simulink model "Simscape_Actuated_Robot"  (R2025b)
settings: Solver=odeN  StartTime=0.0  StopTime=20  RelTol=1e-1  AbsTol=1e-3
InitFcn:
  | run("init.m");
values from neighbouring files (symbols this model uses):
  B = [0 1 0; 1 0 0; 0 0 1; 0 0 0]    [init.m]
  q_init = zeros(6,1)    [init.m]
  s = de + c.*e    [wbr_ctrl.m]
  Ts = 1e-4    (= 0.0001)    [init.m]
undefined symbols (not defined in the file or in its folder): K, robot_params, X, Y, Z
libraries: nesl_utility x53, sm_lib x52, simulink x1
(part 1 of 2)
settings Model: Creator=Acer  LastModifiedBy=Acer
settings SolverCC: AutoScaleAbsTol=off  ODENIntegrationMethod=ode8

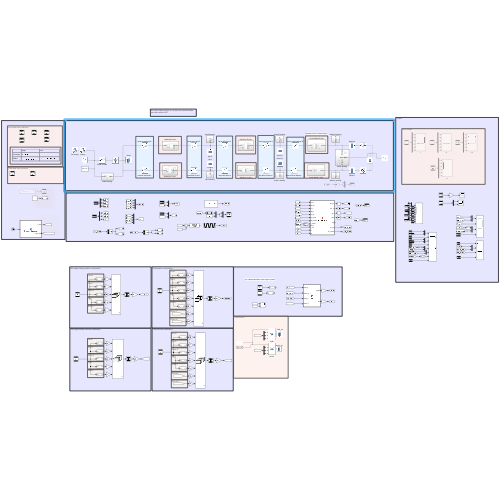
[thumbnail: Simulink's stored preview of the top-level diagram]
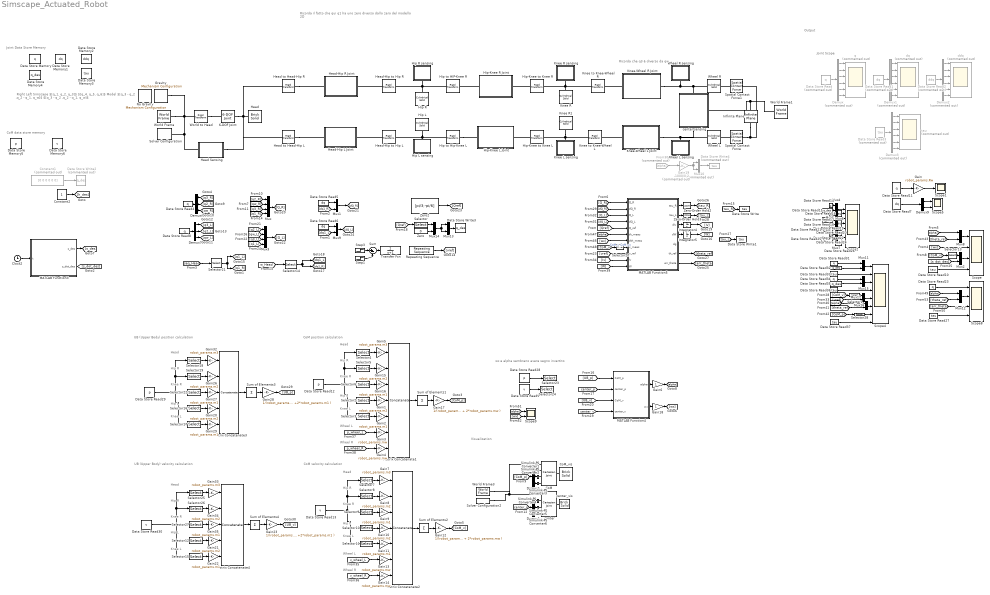
== system Simscape_Actuated_Robot ==
  note: Ricorda che q3 è diverso da qw
  note: wx e alpha sembrano avere segno invertito
  note: Visualization
  note: CoM data store memory
  note: CoM position calculation
  note: ​
      | Right
      | Left
      |
      | Simscape
      | $[q_1, q_2, q_3]$
      | $[q_4, q_5, q_6]$
      |
      | Model
      | $[q_3 - q_2 ,q_2 - q_1, q_w]$
      | $[q_3 - q_2 ,q_2 - q_1, q_w]$
  note: Joint Data Store Memory
  note: Joint Scope
  note: Output
  note: Ricorda il fatto che qui q1 ha uno zero diverso dallo
      | zero del modello 2D
  note: Head
  note: CoM velocity calculation
  note: Hip R
  note: Knee R
  note: Hip L
  note: Knee L
  note: Wheel L
  note: Wheel R
  note: Wheel L
  note: Wheel R
  note: Head
  note: Knee L
  note: Hip R
  note: Knee R
  note: Hip L
  note: UB (Upper Body) position calculation
  note: Head
  note: UB (Upper Body) velocity calculation
  note: Hip R
  note: Knee R
  note: Hip L
  note: Knee L
  note: Head
  note: Knee L
  note: Hip R
  note: Knee R
  note: Hip L
  6-DOF Joint : sm_lib/Joints/6-DOF Joint  JointMode=Normal  CompositeWrenchDir=FollowerOnBase  CompositeWrenchFrame=BaseFrame  SenseConstraintForce=off  SenseConstraintTorque=off  SenseTotalForce=off  SenseTotalTorque=off  PxPositionTargetSpecify=off  PxPositionTargetPriority=High  PxPositionTargetValue=0  PxPositionTargetValueUnits=m  PxVelocityTargetSpecify=off  PxVelocityTargetPriority=High  PxVelocityTargetValue=0  PxVelocityTargetValueUnits=m/s  PxEquilibriumPosition=0  PxEquilibriumPositionUnits=m  PxSpringStiffness=0  PxSpringStiffnessUnits=N/m  PxDampingCoefficient=0  PxDampingCoefficientUnits=N/(m/s)  PxLowerLimitSpecify=off  PxLowerLimitBound=-1  PxLowerLimitBoundUnits=m  PxLowerLimitStiffness=1e6  PxLowerLimitStiffnessUnits=N/m  PxLowerLimitDamping=1e3  PxLowerLimitDampingUnits=N/(m/s)  PxLowerLimitTransitionRegionWidth=1e-4  PxLowerLimitTransitionRegionWidthUnits=m  PxUpperLimitSpecify=off  PxUpperLimitBound=1  PxUpperLimitBoundUnits=m  PxUpperLimitStiffness=1e6  PxUpperLimitStiffnessUnits=N/m  PxUpperLimitDamping=1e3  PxUpperLimitDampingUnits=N/(m/s)  PxUpperLimitTransitionRegionWidth=1e-4  PxUpperLimitTransitionRegionWidthUnits=m  PxTorqueActuationMode=NoTorque  PxMotionActuationMode=ComputedMotion  PxSensePosition=off  PxSenseVelocity=off  PxSenseAcceleration=off  PxSenseTorqueForce=off  PxSenseLowerLimitTorqueForce=off  PxSenseUpperLimitTorqueForce=off  PyPositionTargetSpecify=off  PyPositionTargetPriority=High  PyPositionTargetValue=0  PyPositionTargetValueUnits=m  PyVelocityTargetSpecify=off  PyVelocityTargetPriority=High  PyVelocityTargetValue=0  PyVelocityTargetValueUnits=m/s  PyEquilibriumPosition=0  PyEquilibriumPositionUnits=m  PySpringStiffness=0  PySpringStiffnessUnits=N/m  PyDampingCoefficient=0  PyDampingCoefficientUnits=N/(m/s)  PyLowerLimitSpecify=off  PyLowerLimitBound=-1  PyLowerLimitBoundUnits=m  PyLowerLimitStiffness=1e6  PyLowerLimitStiffnessUnits=N/m  PyLowerLimitDamping=1e3  PyLowerLimitDampingUnits=N/(m/s)  PyLowerLimitTransitionRegionWidth=1e-4  PyLowerLimitTransitionRegionWidthUnits=m  PyUpperLimitSpecify=off  PyUpperLimitBound=1  PyUpperLimitBoundUnits=m  PyUpperLimitStiffness=1e6  PyUpperLimitStiffnessUnits=N/m  PyUpperLimitDamping=1e3  PyUpperLimitDampingUnits=N/(m/s)  PyUpperLimitTransitionRegionWidth=1e-4  PyUpperLimitTransitionRegionWidthUnits=m  PyTorqueActuationMode=NoTorque  PyMotionActuationMode=ComputedMotion  PySensePosition=off  PySenseVelocity=off  PySenseAcceleration=off  PySenseTorqueForce=off  PySenseLowerLimitTorqueForce=off  PySenseUpperLimitTorqueForce=off  PzPositionTargetSpecify=off  PzPositionTargetPriority=High  PzPositionTargetValue=0  PzPositionTargetValueUnits=m  PzVelocityTargetSpecify=off  PzVelocityTargetPriority=High  PzVelocityTargetValue=0  PzVelocityTargetValueUnits=m/s  PzEquilibriumPosition=0  PzEquilibriumPositionUnits=m  PzSpringStiffness=0  PzSpringStiffnessUnits=N/m  PzDampingCoefficient=0  PzDampingCoefficientUnits=N/(m/s)  PzLowerLimitSpecify=off  PzLowerLimitBound=-1  PzLowerLimitBoundUnits=m  PzLowerLimitStiffness=1e6  PzLowerLimitStiffnessUnits=N/m  PzLowerLimitDamping=1e3  PzLowerLimitDampingUnits=N/(m/s)  PzLowerLimitTransitionRegionWidth=1e-4  PzLowerLimitTransitionRegionWidthUnits=m  PzUpperLimitSpecify=off  PzUpperLimitBound=1  PzUpperLimitBoundUnits=m  PzUpperLimitStiffness=1e6  PzUpperLimitStiffnessUnits=N/m  PzUpperLimitDamping=1e3  PzUpperLimitDampingUnits=N/(m/s)  PzUpperLimitTransitionRegionWidth=1e-4  PzUpperLimitTransitionRegionWidthUnits=m  PzTorqueActuationMode=NoTorque  PzMotionActuationMode=ComputedMotion  PzSensePosition=off  PzSenseVelocity=off  PzSenseAcceleration=off  PzSenseTorqueForce=off  PzSenseLowerLimitTorqueForce=off  PzSenseUpperLimitTorqueForce=off  SphPositionTargetSpecify=off  SphPositionTargetPriority=High  SphPositionTargetRotationMethod=None  SphPositionTargetFollAlignAxisA=+X  SphPositionTargetBaseAlignAxisA=+Y  SphPositionTargetFollAlignAxisB=+Y  SphPositionTargetBaseAlignAxisB=+Z  SphPositionTargetRotationStandardAxis=+Z  SphPositionTargetRotationAngle=0  SphPositionTargetRotationAngleUnits=deg  SphPositionTargetRotationArbitraryAxis=[0 0 1]  SphPositionTargetRotationSequenceAxes=FollowerAxes  SphPositionTargetRotationSequence=XYX  SphPositionTargetRotationSequenceAngles=[0 0 0]  SphPositionTargetRotationSequenceAnglesUnits=deg  SphPositionTargetRotationMatrix=[1 0 0;0 1 0;0 0 1]  SphPositionTargetQuaternion=[1 0 0 0]  SphVelocityTargetSpecify=off  SphVelocityTargetPriority=High  SphVelocityTargetValue=[0 0 0]  SphVelocityTargetValueUnits=deg/s  SphVelocityTargetInFollowerFrame=on  SphEqPosRotationMethod=None  SphEqPosFollAlignAxisA=+X  SphEqPosBaseAlignAxisA=+Y  SphEqPosFollAlignAxisB=+Y  SphEqPosBaseAlignAxisB=+Z  SphEqPosRotationStandardAxis=+Z  SphEqPosRotationAngle=0  SphEqPosRotationAngleUnits=deg  SphEqPosRotationArbitraryAxis=[0 0 1]  SphEqPosRotationSequenceAxes=FollowerAxes  SphEqPosRotationSequence=XYX  SphEqPosRotationSequenceAngles=[0 0 0]  SphEqPosRotationSequenceAnglesUnits=deg  SphEqPosRotationMatrix=[1 0 0;0 1 0;0 0 1]  SphEqPosQuaternion=[1 0 0 0]  SphSpringStiffness=0  SphSpringStiffnessUnits=N*m/deg  SphDampingCoefficient=0  SphDampingCoefficientUnits=N*m/(deg/s)  SphLowerLimitSpecify=off  SphLowerLimitBound=15  SphLowerLimitBoundUnits=deg  SphLowerLimitStiffness=1e4  SphLowerLimitStiffnessUnits=N*m/deg  SphLowerLimitDamping=10  SphLowerLimitDampingUnits=N*m/(deg/s)  SphLowerLimitTransitionRegionWidth=0.1  SphLowerLimitTransitionRegionWidthUnits=deg  SphUpperLimitSpecify=off  SphUpperLimitBound=45  SphUpperLimitBoundUnits=deg  SphUpperLimitStiffness=1e4  SphUpperLimitStiffnessUnits=N*m/deg  SphUpperLimitDamping=10  SphUpperLimitDampingUnits=N*m/(deg/s)  SphUpperLimitTransitionRegionWidth=0.1  SphUpperLimitTransitionRegionWidthUnits=deg  SphTorqueActuationMode=NoTorque  SphActuateTorqueX=off  SphActuateTorqueY=off  SphActuateTorqueZ=off  SphActuateTorque=off  SphActuationFrame=BaseFrame  SphSensePosition=off  SphSenseVelocityX=off  SphSenseVelocityY=off  SphSenseVelocityZ=off  SphSenseVelocity=off  SphSenseAccelerationX=off  SphSenseAccelerationY=off  SphSenseAccelerationZ=off  SphSenseAcceleration=off  SphSenseLowerLimitTorqueMag=off  SphSenseUpperLimitTorqueMag=off  SphSensingFrame=BaseFrame
  Clock2 : Clock
  CoM : sm_lib/Joints/Cartesian Joint  JointMode=Normal  CompositeWrenchDir=FollowerOnBase  CompositeWrenchFrame=BaseFrame  SenseConstraintForce=off  SenseConstraintTorque=off  SenseTotalForce=off  SenseTotalTorque=off  PxPositionTargetSpecify=off  PxPositionTargetPriority=High  PxPositionTargetValue=0  PxPositionTargetValueUnits=m  PxVelocityTargetSpecify=off  PxVelocityTargetPriority=High  PxVelocityTargetValue=0  PxVelocityTargetValueUnits=m/s  PxEquilibriumPosition=0  PxEquilibriumPositionUnits=m  PxSpringStiffness=0  PxSpringStiffnessUnits=N/m  PxDampingCoefficient=0  PxDampingCoefficientUnits=N/(m/s)  PxLowerLimitSpecify=off  PxLowerLimitBound=-1  PxLowerLimitBoundUnits=m  PxLowerLimitStiffness=1e6  PxLowerLimitStiffnessUnits=N/m  PxLowerLimitDamping=1e3  PxLowerLimitDampingUnits=N/(m/s)  PxLowerLimitTransitionRegionWidth=1e-4  PxLowerLimitTransitionRegionWidthUnits=m  PxUpperLimitSpecify=off  PxUpperLimitBound=1  PxUpperLimitBoundUnits=m  PxUpperLimitStiffness=1e6  PxUpperLimitStiffnessUnits=N/m  PxUpperLimitDamping=1e3  PxUpperLimitDampingUnits=N/(m/s)  PxUpperLimitTransitionRegionWidth=1e-4  PxUpperLimitTransitionRegionWidthUnits=m  PxTorqueActuationMode=ComputedTorque  PxMotionActuationMode=InputMotion  PxSensePosition=off  PxSenseVelocity=off  PxSenseAcceleration=off  PxSenseTorqueForce=off  PxSenseLowerLimitTorqueForce=off  PxSenseUpperLimitTorqueForce=off  PyPositionTargetSpecify=off  PyPositionTargetPriority=High  PyPositionTargetValue=0  PyPositionTargetValueUnits=m  PyVelocityTargetSpecify=off  PyVelocityTargetPriority=High  PyVelocityTargetValue=0  PyVelocityTargetValueUnits=m/s  PyEquilibriumPosition=0  PyEquilibriumPositionUnits=m  PySpringStiffness=0  PySpringStiffnessUnits=N/m  PyDampingCoefficient=0  PyDampingCoefficientUnits=N/(m/s)  PyLowerLimitSpecify=off  PyLowerLimitBound=-1  PyLowerLimitBoundUnits=m  PyLowerLimitStiffness=1e6  PyLowerLimitStiffnessUnits=N/m  PyLowerLimitDamping=1e3  PyLowerLimitDampingUnits=N/(m/s)  PyLowerLimitTransitionRegionWidth=1e-4  PyLowerLimitTransitionRegionWidthUnits=m  PyUpperLimitSpecify=off  PyUpperLimitBound=1  PyUpperLimitBoundUnits=m  PyUpperLimitStiffness=1e6  PyUpperLimitStiffnessUnits=N/m  PyUpperLimitDamping=1e3  PyUpperLimitDampingUnits=N/(m/s)  PyUpperLimitTransitionRegionWidth=1e-4  PyUpperLimitTransitionRegionWidthUnits=m  PyTorqueActuationMode=ComputedTorque  PyMotionActuationMode=InputMotion  PySensePosition=off  PySenseVelocity=off  PySenseAcceleration=off  PySenseTorqueForce=off  PySenseLowerLimitTorqueForce=off  PySenseUpperLimitTorqueForce=off  PzPositionTargetSpecify=off  PzPositionTargetPriority=High  PzPositionTargetValue=0  PzPositionTargetValueUnits=m  PzVelocityTargetSpecify=off  PzVelocityTargetPriority=High  PzVelocityTargetValue=0  PzVelocityTargetValueUnits=m/s  PzEquilibriumPosition=0  PzEquilibriumPositionUnits=m  PzSpringStiffness=0  PzSpringStiffnessUnits=N/m  PzDampingCoefficient=0  PzDampingCoefficientUnits=N/(m/s)  PzLowerLimitSpecify=off  PzLowerLimitBound=-1  PzLowerLimitBoundUnits=m  PzLowerLimitStiffness=1e6  PzLowerLimitStiffnessUnits=N/m  PzLowerLimitDamping=1e3  PzLowerLimitDampingUnits=N/(m/s)  PzLowerLimitTransitionRegionWidth=1e-4  PzLowerLimitTransitionRegionWidthUnits=m  PzUpperLimitSpecify=off  PzUpperLimitBound=1  PzUpperLimitBoundUnits=m  PzUpperLimitStiffness=1e6  PzUpperLimitStiffnessUnits=N/m  PzUpperLimitDamping=1e3  PzUpperLimitDampingUnits=N/(m/s)  PzUpperLimitTransitionRegionWidth=1e-4  PzUpperLimitTransitionRegionWidthUnits=m  PzTorqueActuationMode=ComputedTorque  PzMotionActuationMode=InputMotion  PzSensePosition=off  PzSenseVelocity=off  PzSenseAcceleration=off  PzSenseTorqueForce=off  PzSenseLowerLimitTorqueForce=off  PzSenseUpperLimitTorqueForce=off
  CoM_vis : sm_lib/Body Elements/Brick Solid  BrickDimensions=[.05 .05 .05]  BrickDimensionsUnits=m  ExportEntireGeometry=off  InertiaType=PointMass  BasedOnType=Density  Density=1000  DensityUnits=kg/m^3  Mass=0.001  MassUnits=kg  CenterOfMass=[0 0 0]  CenterOfMassUnits=m  MomentsOfInertia=[1 1 1]  MomentsOfInertiaUnits=kg*m^2  ProductsOfInertia=[0 0 0]  ProductsOfInertiaUnits=kg*m^2  GraphicType=FromGeometry  MarkerShape=Sphere  MarkerSize=10  GraphicVisPropType=SimpleVisualProperties  GraphicDiffuseColor=[0 0 0]  GraphicOpacity=1  GraphicSpecularColor=[0.5 0.5 0.5 1.0]  GraphicAmbientColor=[0.15 0.15 0.15 1.0]  GraphicEmissiveColor=[0.0 0.0 0.0 1.0]  GraphicShininess=75  DoExposeReferenceFrame=on  SerializedFrames=<Frames/>
  Constant1 : Constant  Commented=on  Value=[0 0 0 0 0 0]
  Constant2 : Constant
  Data Store Memory : DataStoreMemory  Priority=1  DataStoreName=q  WriteAfterWriteMsg=warning  InitialValue=q_init  ShareAcrossModelInstances=on  ShowAdditionalParam=off  OutDataTypeStr=double
  Data Store Memory1 : DataStoreMemory  Priority=2  DataStoreName=dq  WriteAfterWriteMsg=warning  InitialValue=zeros(6,1)  ShareAcrossModelInstances=on  ShowAdditionalParam=off  OutDataTypeStr=double
  Data Store Memory2 : DataStoreMemory  Priority=2  DataStoreName=ddq  WriteAfterWriteMsg=warning  InitialValue=zeros(6,1)  ShareAcrossModelInstances=on  ShowAdditionalParam=off  OutDataTypeStr=double
  Data Store Memory3 : DataStoreMemory  Priority=2  DataStoreName=tau  WriteAfterWriteMsg=warning  InitialValue=zeros(6,1)  ShareAcrossModelInstances=on  ShowAdditionalParam=off  OutDataTypeStr=double
  Data Store Memory4 : DataStoreMemory  DataStoreName=q_des  WriteAfterWriteMsg=warning  InitialValue=zeros(6,1)  ShareAcrossModelInstances=on  ShowAdditionalParam=off  OutDataTypeStr=double
  Data Store Memory5 : DataStoreMemory  Priority=2  DataStoreName=p  WriteAfterWriteMsg=warning  InitialValue=zeros(3,5)  ShareAcrossModelInstances=on  ShowAdditionalParam=off  OutDataTypeStr=double
  Data Store Memory6 : DataStoreMemory  Priority=2  DataStoreName=v  WriteAfterWriteMsg=warning  InitialValue=zeros(3,5)  ShareAcrossModelInstances=on  ShowAdditionalParam=off  OutDataTypeStr=double
  Data Store Read : DataStoreRead  Commented=on  DataStoreName=q  IndexOptions=Index vector (dialog)  Indices=1  OutputSizes=1
  Data Store Read1 : DataStoreRead  Commented=on  DataStoreName=dq  IndexOptions=Index vector (dialog)  Indices=1  OutputSizes=1
  Data Store Read10 : DataStoreRead  DataStoreName=tau  DataStoreElements=tau  EnableIndexing=on  IndexOptions=Index vector (dialog)  Indices=[3 6]  OutputSizes=1
  Data Store Read11 : DataStoreRead  DataStoreName=q  DataStoreElements=q  EnableIndexing=on  IndexOptions=Index vector (dialog)  Indices=[3]  OutputSizes=1
  Data Store Read12 : DataStoreRead  DataStoreName=p  IndexOptions=Index vector (dialog)  Indices=1  OutputSizes=1
  Data Store Read13 : DataStoreRead  DataStoreName=v  IndexOptions=Index vector (dialog)  Indices=1  OutputSizes=1
  Data Store Read14 : DataStoreRead  DataStoreName=q  DataStoreElements=q  EnableIndexing=on  IndexOptions=Index vector (dialog)  Indices=1  OutputSizes=1
  Data Store Read15 : DataStoreRead  DataStoreName=q_des  DataStoreElements=q_des  EnableIndexing=on  IndexOptions=Index vector (dialog)  Indices=[1]  OutputSizes=1
  Data Store Read16 : DataStoreRead  DataStoreName=tau  DataStoreElements=tau  EnableIndexing=on  IndexOptions=Index vector (dialog)  Indices=1  OutputSizes=1
  Data Store Read17 : DataStoreRead  DataStoreName=q  DataStoreElements=q  EnableIndexing=on  IndexOptions=Index vector (dialog)  Indices=2  OutputSizes=1
  Data Store Read18 : DataStoreRead  DataStoreName=q_des  DataStoreElements=q_des  EnableIndexing=on  IndexOptions=Index vector (dialog)  Indices=[2]  OutputSizes=1
  Data Store Read19 : DataStoreRead  DataStoreName=tau  DataStoreElements=tau  EnableIndexing=on  IndexOptions=Index vector (dialog)  Indices=2  OutputSizes=1
  Data Store Read2 : DataStoreRead  Commented=on  DataStoreName=ddq  IndexOptions=Index vector (dialog)  Indices=1  OutputSizes=1
  Data Store Read20 : DataStoreRead  DataStoreName=q  DataStoreElements=q  EnableIndexing=on  IndexOptions=Index vector (dialog)  Indices=4  OutputSizes=1
  Data Store Read21 : DataStoreRead  DataStoreName=q_des  DataStoreElements=q_des  EnableIndexing=on  IndexOptions=Index vector (dialog)  Indices=4  OutputSizes=1
  Data Store Read22 : DataStoreRead  DataStoreName=tau  DataStoreElements=tau  EnableIndexing=on  IndexOptions=Index vector (dialog)  Indices=4  OutputSizes=1
  Data Store Read23 : DataStoreRead  DataStoreName=q  EnableIndexing=on  IndexOptions=Index vector (dialog)  Indices=[3 6]  OutputSizes=1
  Data Store Read24 : DataStoreRead  DataStoreName=q  DataStoreElements=q  EnableIndexing=on  IndexOptions=Index vector (dialog)  Indices=5  OutputSizes=1
  Data Store Read25 : DataStoreRead  DataStoreName=q_des  DataStoreElements=q_des  EnableIndexing=on  IndexOptions=Index vector (dialog)  Indices=5  OutputSizes=1
  Data Store Read26 : DataStoreRead  DataStoreName=tau  DataStoreElements=tau  EnableIndexing=on  IndexOptions=Index vector (dialog)  Indices=5  OutputSizes=1
  Data Store Read27 : DataStoreRead  DataStoreName=tau  DataStoreElements=tau  EnableIndexing=on  IndexOptions=Index vector (dialog)  Indices=[3 6]  OutputSizes=1
  Data Store Read28 : DataStoreRead  DataStoreName=p  IndexOptions=Index vector (dialog)  Indices=1  OutputSizes=1
  Data Store Read29 : DataStoreRead  DataStoreName=p  IndexOptions=Index vector (dialog)  Indices=1  OutputSizes=1
  Data Store Read3 : DataStoreRead  Commented=on  DataStoreName=tau  IndexOptions=Index vector (dialog)  Indices=1  OutputSizes=1
  Data Store Read30 : DataStoreRead  DataStoreName=v  IndexOptions=Index vector (dialog)  Indices=1  OutputSizes=1
  Data Store Read31 : DataStoreRead  DataStoreName=q  DataStoreElements=q  EnableIndexing=on  IndexOptions=Index vector (dialog)  Indices=1  OutputSizes=1
  Data Store Read32 : DataStoreRead  DataStoreName=q_des  DataStoreElements=q_des  EnableIndexing=on  IndexOptions=Index vector (dialog)  Indices=[1]  OutputSizes=1
  Data Store Read33 : DataStoreRead  DataStoreName=tau  DataStoreElements=tau  EnableIndexing=on  IndexOptions=Index vector (dialog)  Indices=1  OutputSizes=1
  Data Store Read34 : DataStoreRead  DataStoreName=q  DataStoreElements=q  EnableIndexing=on  IndexOptions=Index vector (dialog)  Indices=2  OutputSizes=1
  Data Store Read35 : DataStoreRead  DataStoreName=q_des  DataStoreElements=q_des  EnableIndexing=on  IndexOptions=Index vector (dialog)  Indices=[2]  OutputSizes=1
  Data Store Read36 : DataStoreRead  DataStoreName=tau  DataStoreElements=tau  EnableIndexing=on  IndexOptions=Index vector (dialog)  Indices=2  OutputSizes=1
  Data Store Read37 : DataStoreRead  DataStoreName=tau  DataStoreElements=tau  EnableIndexing=on  IndexOptions=Index vector (dialog)  Indices=[3 6]  OutputSizes=1
  Data Store Read4 : DataStoreRead  DataStoreName=q  DataStoreElements=q  EnableIndexing=on  IndexOptions=Index vector (dialog)  Indices=[1 2 3]  OutputSizes=1
  Data Store Read5 : DataStoreRead  DataStoreName=dq  DataStoreElements=dq  EnableIndexing=on  IndexOptions=Index vector (dialog)  Indices=[2 3 1]  OutputSizes=1
  Data Store Read6 : DataStoreRead  DataStoreName=dq  DataStoreElements=dq  EnableIndexing=on  IndexOptions=Index vector (dialog)  Indices=[5 6 4]  OutputSizes=1
  Data Store Read7 : DataStoreRead  DataStoreName=dq  DataStoreElements=dq  EnableIndexing=on  IndexOptions=Index vector (dialog)  Indices=[3, 6]  OutputSizes=1
  Data Store Read8 : DataStoreRead  DataStoreName=q  DataStoreElements=q  EnableIndexing=on  IndexOptions=Index vector (dialog)  Indices=[4 5 6]  OutputSizes=1
  Data Store Read9 : DataStoreRead  DataStoreName=v  IndexOptions=Index vector (dialog)  Indices=1  OutputSizes=1
  Data Store Write : DataStoreWrite  DataStoreName=tau  DataStoreElements=tau  EnableIndexing=on  IndexOptions=Index vector (dialog)  Indices=[3 2 1]  OutputSizes=1
  Data Store Write1 : DataStoreWrite  DataStoreName=tau  DataStoreElements=tau  EnableIndexing=on  IndexOptions=Index vector (dialog)  Indices=[6 5 4]  OutputSizes=1
  Data Store Write2 : DataStoreWrite  Commented=on  DataStoreName=q_des  IndexOptions=Index vector (dialog)  Indices=1  OutputSizes=1
  Data Store Write3 : DataStoreWrite  DataStoreName=q_des  IndexOptions=Index vector (dialog)  Indices=1  OutputSizes=1
  Data Store Write4 : DataStoreWrite  Commented=on  DataStoreName=tau  DataStoreElements=tau  EnableIndexing=on  IndexOptions=Index vector (dialog)  Indices=[3 6]  OutputSizes=1
  Demux{,1..3} (4 alike) : Demux  Commented=on  Outputs=6
  Demux{4..7} (4 alike) : Demux  Outputs=3
  Demux9 : Demux  Outputs=2
  From30 : From  Commented=on  GotoTag=alpha
  Gain : Gain  Gain=robot_params.Rw
  Gain{1,8,10,15,20..21,26,34} (8 alike) : Gain  Gain=robot_params.m2
  Gain{2,9,11,16,22,27,29,35} (8 alike) : Gain  Gain=robot_params.m1
  Gain12 : Gain  Gain=1/(robot_params.m3 + 2*robot_params.m2 +2*robot_params.m1 + 2*robot_params.mw )
  Gain{3..4,13..14} (4 alike) : Gain  Gain=robot_params.mw
  Gain17 : Gain  Gain=1/(robot_params.m3 + 2*robot_params.m2 +2*robot_params.m1 + 2*robot_params.mw )
  Gain18 : Gain
  Gain19 : Gain  Commented=on  Gain=-1000/0.2
  Gain23 : Gain  Gain=1/(robot_params.m3 + 2*robot_params.m2 +2*robot_params.m1 )
  Gain28 : Gain  Gain=1/(robot_params.m3 + 2*robot_params.m2 +2*robot_params.m1 )
  Gain{5,7,32..33} (4 alike) : Gain  Gain=robot_params.m3
  Gain6 : Gain
  Gravity : sm_lib/Utilities/Mechanism Configuration  UniformGravity=Constant  GravityVector=[0 0 -9.80665]  GravityVectorUnits=m/s^2  LinearizationDelta=0.001  JointModeTransitionNonlinearIterations=2
  Head : sm_lib/Body Elements/Brick Solid  BrickDimensions=robot_params.length_torso  BrickDimensionsUnits=m  ExportEntireGeometry=off  InertiaType=Custom  BasedOnType=Density  Density=1000  DensityUnits=kg/m^3  Mass=robot_params.m3  MassUnits=kg  CenterOfMass=[0 0 0]  CenterOfMassUnits=m  MomentsOfInertia=robot_params.inertia_torso  MomentsOfInertiaUnits=kg*m^2  ProductsOfInertia=[0 0 0]  ProductsOfInertiaUnits=kg*m^2  GraphicType=FromGeometry  MarkerShape=Sphere  MarkerSize=10  GraphicVisPropType=SimpleVisualProperties  GraphicDiffuseColor=[0.5 0.5 0.5]  GraphicOpacity=1  GraphicSpecularColor=[0.5 0.5 0.5 1.0]  GraphicAmbientColor=[0.15 0.15 0.15 1.0]  GraphicEmissiveColor=[0.0 0.0 0.0 1.0]  GraphicShininess=75  DoExposeReferenceFrame=on  SerializedFrames=<Frames/>
  Head Sensing : Subsystem
  "Head to Head-Hip L " : sm_lib/Frames and Transforms/Rigid Transform  RotationMethod=RotationSequence  FollAlignAxisA=+X  BaseAlignAxisA=+Y  FollAlignAxisB=+Y  BaseAlignAxisB=+Z  RotationStandardAxis=+Z  RotationAngle=0  RotationAngleUnits=deg  RotationArbitraryAxis=[0 0 1]  RotationSequenceAxes=FollowerAxes  RotationSequence=XYZ  RotationSequenceAngles=[pi/2 0 0]  RotationSequenceAnglesUnits=rad  RotationMatrix=[1 0 0;0 1 0;0 0 1]  Quaternion=[1 0 0 0]  TranslationMethod=Cartesian  TranslationCartesianOffset=[0 -63/2 -35/2]  TranslationCartesianOffsetUnits=cm  TranslationStandardAxis=+Z  TranslationStandardOffset=0  TranslationStandardOffsetUnits=m  TranslationROffset=0  TranslationROffsetUnits=m  TranslationThetaOffset=0  TranslationThetaOffsetUnits=deg  TranslationZOffset=0  TranslationZOffsetUnits=m
  "Head to Head-Hip R  " : sm_lib/Frames and Transforms/Rigid Transform  RotationMethod=RotationSequence  FollAlignAxisA=+X  BaseAlignAxisA=+Y  FollAlignAxisB=+Y  BaseAlignAxisB=+Z  RotationStandardAxis=+Z  RotationAngle=0  RotationAngleUnits=deg  RotationArbitraryAxis=[0 0 1]  RotationSequenceAxes=FollowerAxes  RotationSequence=XYZ  RotationSequenceAngles=[pi/2 0 0]  RotationSequenceAnglesUnits=rad  RotationMatrix=[1 0 0;0 1 0;0 0 1]  Quaternion=[1 0 0 0]  TranslationMethod=Cartesian  TranslationCartesianOffset=[0 63/2 -35/2]  TranslationCartesianOffsetUnits=cm  TranslationStandardAxis=+Z  TranslationStandardOffset=0  TranslationStandardOffsetUnits=m  TranslationROffset=0  TranslationROffsetUnits=m  TranslationThetaOffset=0  TranslationThetaOffsetUnits=deg  TranslationZOffset=0  TranslationZOffsetUnits=m
  "Head-Hip L Joint " : Subsystem
  "Head-Hip R Joint " : Subsystem
  Head-Hip to Hip L : sm_lib/Frames and Transforms/Rigid Transform  RotationMethod=RotationSequence  FollAlignAxisA=+X  BaseAlignAxisA=+Y  FollAlignAxisB=+Y  BaseAlignAxisB=+Z  RotationStandardAxis=+Z  RotationAngle=0  RotationAngleUnits=deg  RotationArbitraryAxis=[0 0 1]  RotationSequenceAxes=FollowerAxes  RotationSequence=XYZ  RotationSequenceAngles=[pi/2 0 0]  RotationSequenceAnglesUnits=rad  RotationMatrix=[1 0 0;0 1 0;0 0 1]  Quaternion=[1 0 0 0]  TranslationMethod=Cartesian  TranslationCartesianOffset=[0 -45/2 0]  TranslationCartesianOffsetUnits=cm  TranslationStandardAxis=+Z  TranslationStandardOffset=0  TranslationStandardOffsetUnits=m  TranslationROffset=0  TranslationROffsetUnits=m  TranslationThetaOffset=0  TranslationThetaOffsetUnits=deg  TranslationZOffset=0  TranslationZOffsetUnits=m
  Head-Hip to Hip R : sm_lib/Frames and Transforms/Rigid Transform  RotationMethod=RotationSequence  FollAlignAxisA=+X  BaseAlignAxisA=+Y  FollAlignAxisB=+Y  BaseAlignAxisB=+Z  RotationStandardAxis=+Z  RotationAngle=0  RotationAngleUnits=deg  RotationArbitraryAxis=[0 0 1]  RotationSequenceAxes=FollowerAxes  RotationSequence=XYZ  RotationSequenceAngles=[pi/2 0 0]  RotationSequenceAnglesUnits=rad  RotationMatrix=[1 0 0;0 1 0;0 0 1]  Quaternion=[1 0 0 0]  TranslationMethod=Cartesian  TranslationCartesianOffset=[0 -45/2 0]  TranslationCartesianOffsetUnits=cm  TranslationStandardAxis=+Z  TranslationStandardOffset=0  TranslationStandardOffsetUnits=m  TranslationROffset=0  TranslationROffsetUnits=m  TranslationThetaOffset=0  TranslationThetaOffsetUnits=deg  TranslationZOffset=0  TranslationZOffsetUnits=m
  Hip L : sm_lib/Body Elements/Cylindrical Solid  CylinderRadius=robot_params.radius_coscia  CylinderRadiusUnits=m  CylinderLength=robot_params.l2  CylinderLengthUnits=m  ExportEntireGeometry=off  InertiaType=Custom  BasedOnType=Density  Density=1000  DensityUnits=kg/m^3  Mass=robot_params.m2  MassUnits=kg  CenterOfMass=[0 0 0]  CenterOfMassUnits=m  MomentsOfInertia=robot_params.inertia_coscia  MomentsOfInertiaUnits=kg*m^2  ProductsOfInertia=[0 0 0]  ProductsOfInertiaUnits=kg*m^2  GraphicType=FromGeometry  MarkerShape=Sphere  MarkerSize=10  GraphicVisPropType=SimpleVisualProperties  GraphicDiffuseColor=[0.102 0 0.502]  GraphicOpacity=1  GraphicSpecularColor=[0.5 0.5 0.5 1.0]  GraphicAmbientColor=[0.15 0.15 0.15 1.0]  GraphicEmissiveColor=[0.0 0.0 0.0 1.0]  GraphicShininess=75  DoExposeReferenceFrame=on  SerializedFrames=<Frames/>
  Hip L sensing : Subsystem
      settings: PortSchema="{\"entries\":[{\"content\":{\"sides\":[{\"content\":{},\"type\":\"ConnectorPlacement.EquallySpacedRectSide\",\"uuid\":\"ea9d79d0-a490-4652-82e6-557e12b0aba5\"},{\"content\":{\"side\":\"RIGHT\"},\"type\":\"ConnectorPlacement.EquallySpacedRectSide\",\"uuid\":\"f32903a1-4d8b-4407-8bbb-547edd3cb5f6\"},{\"content\":{\"side\":\"TOP\"},\"type\":\"ConnectorPlacement.EquallySpacedRectSide\",\"uuid\":\"fbee0b4d-6271-40ea-8dd1-d28f8c19f4ef\"},{\"content\":{\"connectorIds\":[\"RConn1\"],\"side\":\"BOTTOM\"},\"type\":\"ConnectorPlacement.EquallySpacedRectSide\",\"uuid\":\"cbab87b1-08d9-47a6-9493-a07b4ae6b609\"}]},\"type\":\"ConnectorPlacement.EquallySpacedConnector\",\"uuid\":\"a82548d1-a5fc-4c9c-b8a0-1d70df1cc0c8\"}],\"packageUris\":[\"http://schema.mathworks.com/mf0/Connector/R2020b\"],\"version\":\"1.0\"}"
  Hip R : sm_lib/Body Elements/Cylindrical Solid  CylinderRadius=robot_params.radius_coscia  CylinderRadiusUnits=m  CylinderLength=robot_params.l2  CylinderLengthUnits=m  ExportEntireGeometry=off  InertiaType=Custom  BasedOnType=Density  Density=1000  DensityUnits=kg/m^3  Mass=robot_params.m2  MassUnits=kg  CenterOfMass=[0 0 0]  CenterOfMassUnits=m  MomentsOfInertia=robot_params.inertia_coscia  MomentsOfInertiaUnits=kg*m^2  ProductsOfInertia=[0 0 0]  ProductsOfInertiaUnits=kg*m^2  GraphicType=FromGeometry  MarkerShape=Sphere  MarkerSize=10  GraphicVisPropType=SimpleVisualProperties  GraphicDiffuseColor=[0.102 0 0.502]  GraphicOpacity=1  GraphicSpecularColor=[0.5 0.5 0.5 1.0]  GraphicAmbientColor=[0.15 0.15 0.15 1.0]  GraphicEmissiveColor=[0.0 0.0 0.0 1.0]  GraphicShininess=75  DoExposeReferenceFrame=on  SerializedFrames=<Frames/>
  Hip R sensing : Subsystem
      settings: PortSchema="{\"entries\":[{\"content\":{\"sides\":[{\"content\":{},\"type\":\"ConnectorPlacement.EquallySpacedRectSide\",\"uuid\":\"ea9d79d0-a490-4652-82e6-557e12b0aba5\"},{\"content\":{\"side\":\"RIGHT\"},\"type\":\"ConnectorPlacement.EquallySpacedRectSide\",\"uuid\":\"f32903a1-4d8b-4407-8bbb-547edd3cb5f6\"},{\"content\":{\"side\":\"TOP\"},\"type\":\"ConnectorPlacement.EquallySpacedRectSide\",\"uuid\":\"fbee0b4d-6271-40ea-8dd1-d28f8c19f4ef\"},{\"content\":{\"connectorIds\":[\"RConn1\"],\"side\":\"BOTTOM\"},\"type\":\"ConnectorPlacement.EquallySpacedRectSide\",\"uuid\":\"cbab87b1-08d9-47a6-9493-a07b4ae6b609\"}]},\"type\":\"ConnectorPlacement.EquallySpacedConnector\",\"uuid\":\"a82548d1-a5fc-4c9c-b8a0-1d70df1cc0c8\"}],\"packageUris\":[\"http://schema.mathworks.com/mf0/Connector/R2020b\"],\"version\":\"1.0\"}"
  "Hip to HIP-Knee R " : sm_lib/Frames and Transforms/Rigid Transform  RotationMethod=RotationSequence  FollAlignAxisA=+X  BaseAlignAxisA=+Y  FollAlignAxisB=+Y  BaseAlignAxisB=+Z  RotationStandardAxis=+Z  RotationAngle=0  RotationAngleUnits=deg  RotationArbitraryAxis=[0 0 1]  RotationSequenceAxes=FollowerAxes  RotationSequence=XYZ  RotationSequenceAngles=[-pi/2 0 0]  RotationSequenceAnglesUnits=rad  RotationMatrix=[1 0 0;0 1 0;0 0 1]  Quaternion=[1 0 0 0]  TranslationMethod=Cartesian  TranslationCartesianOffset=[0 0 45/2]  TranslationCartesianOffsetUnits=cm  TranslationStandardAxis=+Z  TranslationStandardOffset=0  TranslationStandardOffsetUnits=m  TranslationROffset=0  TranslationROffsetUnits=m  TranslationThetaOffset=0  TranslationThetaOffsetUnits=deg  TranslationZOffset=0  TranslationZOffsetUnits=m
  Hip to Hip-Knee L : sm_lib/Frames and Transforms/Rigid Transform  RotationMethod=RotationSequence  FollAlignAxisA=+X  BaseAlignAxisA=+Y  FollAlignAxisB=+Y  BaseAlignAxisB=+Z  RotationStandardAxis=+Z  RotationAngle=0  RotationAngleUnits=deg  RotationArbitraryAxis=[0 0 1]  RotationSequenceAxes=FollowerAxes  RotationSequence=XYZ  RotationSequenceAngles=[-pi/2 0 0]  RotationSequenceAnglesUnits=rad  RotationMatrix=[1 0 0;0 1 0;0 0 1]  Quaternion=[1 0 0 0]  TranslationMethod=Cartesian  TranslationCartesianOffset=[0 0 45/2]  TranslationCartesianOffsetUnits=cm  TranslationStandardAxis=+Z  TranslationStandardOffset=0  TranslationStandardOffsetUnits=m  TranslationROffset=0  TranslationROffsetUnits=m  TranslationThetaOffset=0  TranslationThetaOffsetUnits=deg  TranslationZOffset=0  TranslationZOffsetUnits=m
  Hip-Knee L Joint : Subsystem
  Hip-Knee R Joint : Subsystem
  Hip-Knee to Knee L : sm_lib/Frames and Transforms/Rigid Transform  RotationMethod=RotationSequence  FollAlignAxisA=+X  BaseAlignAxisA=+Y  FollAlignAxisB=+Y  BaseAlignAxisB=+Z  RotationStandardAxis=+Z  RotationAngle=0  RotationAngleUnits=deg  RotationArbitraryAxis=[0 0 1]  RotationSequenceAxes=FollowerAxes  RotationSequence=XYZ  RotationSequenceAngles=[pi/2 0 0]  RotationSequenceAnglesUnits=rad  RotationMatrix=[1 0 0;0 1 0;0 0 1]  Quaternion=[1 0 0 0]  TranslationMethod=Cartesian  TranslationCartesianOffset=[0 -45/2 0]  TranslationCartesianOffsetUnits=cm  TranslationStandardAxis=+Z  TranslationStandardOffset=0  TranslationStandardOffsetUnits=m  TranslationROffset=0  TranslationROffsetUnits=m  TranslationThetaOffset=0  TranslationThetaOffsetUnits=deg  TranslationZOffset=0  TranslationZOffsetUnits=m
  Hip-Knee to Knee R : sm_lib/Frames and Transforms/Rigid Transform  RotationMethod=RotationSequence  FollAlignAxisA=+X  BaseAlignAxisA=+Y  FollAlignAxisB=+Y  BaseAlignAxisB=+Z  RotationStandardAxis=+Z  RotationAngle=0  RotationAngleUnits=deg  RotationArbitraryAxis=[0 0 1]  RotationSequenceAxes=FollowerAxes  RotationSequence=XYZ  RotationSequenceAngles=[pi/2 0 0]  RotationSequenceAnglesUnits=rad  RotationMatrix=[1 0 0;0 1 0;0 0 1]  Quaternion=[1 0 0 0]  TranslationMethod=Cartesian  TranslationCartesianOffset=[0 -45/2 0]  TranslationCartesianOffsetUnits=cm  TranslationStandardAxis=+Z  TranslationStandardOffset=0  TranslationStandardOffsetUnits=m  TranslationROffset=0  TranslationROffsetUnits=m  TranslationThetaOffset=0  TranslationThetaOffsetUnits=deg  TranslationZOffset=0  TranslationZOffsetUnits=m
  Infinite Plane : sm_lib/Curves and Surfaces/Infinite Plane  GraphicType=Rectangle  GraphicPlaneWidth=10  GraphicPlaneWidthUnits=m  GraphicPlaneHeight=10  GraphicPlaneHeightUnits=m  GraphicVisPropType=SimpleVisualProperties  GraphicDiffuseColor=[0.1529 0.502 0.04706]  GraphicOpacity=1  GraphicSpecularColor=[0.5 0.5 0.5 1.0]  GraphicAmbientColor=[0.15 0.15 0.15 1.0]  GraphicEmissiveColor=[0.0 0.0 0.0 1.0]  GraphicShininess=75
  Integrator4 : Integrator
  Integrator5 : Integrator  InitialCondition=[0;0;0]
  Knee L sensing : Subsystem
      settings: PortSchema="{\"entries\":[{\"content\":{\"sides\":[{\"content\":{},\"type\":\"ConnectorPlacement.EquallySpacedRectSide\",\"uuid\":\"ea9d79d0-a490-4652-82e6-557e12b0aba5\"},{\"content\":{\"side\":\"RIGHT\"},\"type\":\"ConnectorPlacement.EquallySpacedRectSide\",\"uuid\":\"f32903a1-4d8b-4407-8bbb-547edd3cb5f6\"},{\"content\":{\"side\":\"TOP\"},\"type\":\"ConnectorPlacement.EquallySpacedRectSide\",\"uuid\":\"fbee0b4d-6271-40ea-8dd1-d28f8c19f4ef\"},{\"content\":{\"connectorIds\":[\"RConn1\"],\"side\":\"BOTTOM\"},\"type\":\"ConnectorPlacement.EquallySpacedRectSide\",\"uuid\":\"cbab87b1-08d9-47a6-9493-a07b4ae6b609\"}]},\"type\":\"ConnectorPlacement.EquallySpacedConnector\",\"uuid\":\"a82548d1-a5fc-4c9c-b8a0-1d70df1cc0c8\"}],\"packageUris\":[\"http://schema.mathworks.com/mf0/Connector/R2020b\"],\"version\":\"1.0\"}"
  Knee R : sm_lib/Body Elements/Cylindrical Solid  CylinderRadius=robot_params.radius_stinco  CylinderRadiusUnits=m  CylinderLength=robot_params.l1  CylinderLengthUnits=m  ExportEntireGeometry=off  InertiaType=Custom  BasedOnType=Density  Density=1000  DensityUnits=kg/m^3  Mass=robot_params.m2  MassUnits=kg  CenterOfMass=[0 0 0]  CenterOfMassUnits=m  MomentsOfInertia=robot_params.inertia_stinco  MomentsOfInertiaUnits=kg*m^2  ProductsOfInertia=[0 0 0]  ProductsOfInertiaUnits=kg*m^2  GraphicType=FromGeometry  MarkerShape=Sphere  MarkerSize=10  GraphicVisPropType=SimpleVisualProperties  GraphicDiffuseColor=[0.7569 0 0]  GraphicOpacity=1  GraphicSpecularColor=[0.5 0.5 0.5 1.0]  GraphicAmbientColor=[0.15 0.15 0.15 1.0]  GraphicEmissiveColor=[0.0 0.0 0.0 1.0]  GraphicShininess=75  DoExposeReferenceFrame=on  SerializedFrames=<Frames/>
  Knee R sensing : Subsystem
      settings: PortSchema="{\"entries\":[{\"content\":{\"sides\":[{\"content\":{},\"type\":\"ConnectorPlacement.EquallySpacedRectSide\",\"uuid\":\"ea9d79d0-a490-4652-82e6-557e12b0aba5\"},{\"content\":{\"side\":\"RIGHT\"},\"type\":\"ConnectorPlacement.EquallySpacedRectSide\",\"uuid\":\"f32903a1-4d8b-4407-8bbb-547edd3cb5f6\"},{\"content\":{\"side\":\"TOP\"},\"type\":\"ConnectorPlacement.EquallySpacedRectSide\",\"uuid\":\"fbee0b4d-6271-40ea-8dd1-d28f8c19f4ef\"},{\"content\":{\"connectorIds\":[\"RConn1\"],\"side\":\"BOTTOM\"},\"type\":\"ConnectorPlacement.EquallySpacedRectSide\",\"uuid\":\"cbab87b1-08d9-47a6-9493-a07b4ae6b609\"}]},\"type\":\"ConnectorPlacement.EquallySpacedConnector\",\"uuid\":\"a82548d1-a5fc-4c9c-b8a0-1d70df1cc0c8\"}],\"packageUris\":[\"http://schema.mathworks.com/mf0/Connector/R2020b\"],\"version\":\"1.0\"}"
  Knee R1 : sm_lib/Body Elements/Cylindrical Solid  CylinderRadius=robot_params.radius_stinco  CylinderRadiusUnits=m  CylinderLength=robot_params.l1  CylinderLengthUnits=m  ExportEntireGeometry=off  InertiaType=Custom  BasedOnType=Density  Density=1000  DensityUnits=kg/m^3  Mass=robot_params.m2  MassUnits=kg  CenterOfMass=[0 0 0]  CenterOfMassUnits=m  MomentsOfInertia=robot_params.inertia_stinco  MomentsOfInertiaUnits=kg*m^2  ProductsOfInertia=[0 0 0]  ProductsOfInertiaUnits=kg*m^2  GraphicType=FromGeometry  MarkerShape=Sphere  MarkerSize=10  GraphicVisPropType=SimpleVisualProperties  GraphicDiffuseColor=[0.7569 0 0]  GraphicOpacity=1  GraphicSpecularColor=[0.5 0.5 0.5 1.0]  GraphicAmbientColor=[0.15 0.15 0.15 1.0]  GraphicEmissiveColor=[0.0 0.0 0.0 1.0]  GraphicShininess=75  DoExposeReferenceFrame=on  SerializedFrames=<Frames/>
  Knee to Knee-Wheel L : sm_lib/Frames and Transforms/Rigid Transform  RotationMethod=RotationSequence  FollAlignAxisA=+X  BaseAlignAxisA=+Y  FollAlignAxisB=+Y  BaseAlignAxisB=+Z  RotationStandardAxis=+Z  RotationAngle=0  RotationAngleUnits=deg  RotationArbitraryAxis=[0 0 1]  RotationSequenceAxes=FollowerAxes  RotationSequence=XYZ  RotationSequenceAngles=[-pi/2 0 0]  RotationSequenceAnglesUnits=rad  RotationMatrix=[1 0 0;0 1 0;0 0 1]  Quaternion=[1 0 0 0]  TranslationMethod=Cartesian  TranslationCartesianOffset=[0 2.5 45/2]  TranslationCartesianOffsetUnits=cm  TranslationStandardAxis=+Z  TranslationStandardOffset=0  TranslationStandardOffsetUnits=m  TranslationROffset=0  TranslationROffsetUnits=m  TranslationThetaOffset=0  TranslationThetaOffsetUnits=deg  TranslationZOffset=0  TranslationZOffsetUnits=m
  "Knee to Knee-Wheel R " : sm_lib/Frames and Transforms/Rigid Transform  RotationMethod=RotationSequence  FollAlignAxisA=+X  BaseAlignAxisA=+Y  FollAlignAxisB=+Y  BaseAlignAxisB=+Z  RotationStandardAxis=+Z  RotationAngle=0  RotationAngleUnits=deg  RotationArbitraryAxis=[0 0 1]  RotationSequenceAxes=FollowerAxes  RotationSequence=XYZ  RotationSequenceAngles=[-pi/2 0 0]  RotationSequenceAnglesUnits=rad  RotationMatrix=[1 0 0;0 1 0;0 0 1]  Quaternion=[1 0 0 0]  TranslationMethod=Cartesian  TranslationCartesianOffset=[0 -2.5 45/2]  TranslationCartesianOffsetUnits=cm  TranslationStandardAxis=+Z  TranslationStandardOffset=0  TranslationStandardOffsetUnits=m  TranslationROffset=0  TranslationROffsetUnits=m  TranslationThetaOffset=0  TranslationThetaOffsetUnits=deg  TranslationZOffset=0  TranslationZOffsetUnits=m
  Knee-Wheel L Joint : Subsystem
  Knee-Wheel R Joint : Subsystem
  MATLAB Function3 : MATLAB Function  TreatAsAtomicUnit=on
  MATLAB Function4 : MATLAB Function  TreatAsAtomicUnit=on
  MATLAB Function5 : MATLAB Function  TreatAsAtomicUnit=on
  Matrix Concatenate1 : Concatenate  NumInputs=7  Mode=Multidimensional array  ConcatenateDimension=2
  Matrix Concatenate2 : Concatenate  NumInputs=7  Mode=Multidimensional array  ConcatenateDimension=2
  Matrix Concatenate3 : Concatenate  NumInputs=5  Mode=Multidimensional array  ConcatenateDimension=2
  Matrix Concatenate4 : Concatenate  NumInputs=5  Mode=Multidimensional array  ConcatenateDimension=2
  Mux : Mux
  Mux1 : Mux  Inputs=[3 1]
  Mux10 : Mux  Commented=on  Inputs=2
  Mux{2,4..8,11..13,15..17} (12 alike) : Mux  Inputs=2
  Mux14 : Mux  Inputs=[2 1]
  Mux3 : Mux
  Mux9 : Mux  Inputs=[3 1]
  No Gravity : sm_lib/Utilities/Mechanism Configuration  UniformGravity=Constant  GravityVector=[0 0 0]  GravityVectorUnits=m/s^2  LinearizationDelta=0.001  JointModeTransitionNonlinearIterations=2
  Repeating Sequence : simulink/Sources/Repeating Sequence  rep_seq_t=[0 1 3 5.5 7.5 8 10 ]  rep_seq_y=[0 0 -0.25 -0.25 0 0 0]
  Scope : Scope  NumInputPorts=4
      settings: ActiveDisplayString=4  Title=tau wheel  ActiveDisplayYMinimum=-282.80634407867814  ActiveDisplayYMaximum=45.257096708103127  DataLoggingVariableName=ScopeData5
  Scope1 : Scope
      settings: ActiveDisplayYMinimum=-0.23778714291347786  ActiveDisplayYMaximum=2.0522699916124849  DataLoggingVariableName=ScopeData4
  Scope2 : Scope  NumInputPorts=8
      settings: TimeSpan=1  ActiveDisplayString=3  Title=q ginocchio R  ActiveDisplayYMinimum=-0.34760251692200972  ActiveDisplayYMaximum=1.2021753365431096  DataLoggingVariableName=ScopeData6
  Scope4 : Scope  NumInputPorts=8
      settings: TimeSpan=1  ActiveDisplayString=7  Title=CoM_pos  ActiveDisplayYMinimum=-1.8815644307433808  ActiveDisplayYMaximum=0.23334218779246438  DataLoggingVariableName=ScopeData8
  Scope5 : Scope  NumInputPorts=2
      settings: Title=dqw R  ActiveDisplayYMinimum=-1.3835417658805529  ActiveDisplayYMaximum=1.5686236558627678  DataLoggingVariableName=ScopeData9
  Scope8 : Scope  NumInputPorts=4
      settings: ActiveDisplayString=4  Title=tau wheel  ActiveDisplayYMinimum=-59.873273907276818  ActiveDisplayYMaximum=84.0339033515749  DataLoggingVariableName=ScopeData12
  Scope9 : Scope  NumInputPorts=2
      settings: Title=wx  ActiveDisplayYMinimum=-3.5349420932219275  ActiveDisplayYMaximum=0.965450587960937  DataLoggingVariableName=ScopeData13
  Selector : Selector  InputPortWidth=2  IndexOptions=Index vector (dialog)  Indices=[2 1]  OutputSizes=1
  Selector{1,13,20,28} (4 alike) : Selector  InputPortWidth=3  IndexOptions=Index vector (dialog)  Indices=[1]  OutputSizes=1
  Selector{2,10,12,16} (4 alike) : Selector  NumberOfDimensions=2  InputPortWidth=3  IndexOptions=Index vector (dialog),Index vector (dialog)  Indices=[1 2 3],[4]  OutputSizes=1,1
  Selector{3,11,15,17} (4 alike) : Selector  NumberOfDimensions=2  InputPortWidth=3  IndexOptions=Index vector (dialog),Index vector (dialog)  Indices=[1 2 3],[5]  OutputSizes=1,1
  Selector14 : Selector  InputPortWidth=3  IndexOptions=Index vector (dialog)  Indices=[2]  OutputSizes=1
  Selector{4,7,18,23..25} (6 alike) : Selector  NumberOfDimensions=2  InputPortWidth=3  IndexOptions=Index vector (dialog),Index vector (dialog)  Indices=[1 2 3],[1]  OutputSizes=1,1
  Selector{5,8,19,26} (4 alike) : Selector  NumberOfDimensions=2  InputPortWidth=3  IndexOptions=Index vector (dialog),Index vector (dialog)  Indices=[1 2 3],[2]  OutputSizes=1,1
  Selector21 : Selector  InputPortWidth=3  IndexOptions=Index vector (dialog)  Indices=[2]  OutputSizes=1
  Selector{6,9,22,27} (4 alike) : Selector  NumberOfDimensions=2  InputPortWidth=3  IndexOptions=Index vector (dialog),Index vector (dialog)  Indices=[1 2 3],[3]  OutputSizes=1,1
  Simulink-PS Converter{1..6} (6 alike) : nesl_utility/Simulink-PS Converter  PhysicalDomain=network_engine_domain  SubClassName=ps_input  LeftPortType=input  RightPortType=output  PseudoPeriodic=off  Frequencies=[]  NoiseDistribution=none  NoiseParameters=[]  Unit=1  AffineConversion=off  FilteringAndDerivatives=zero  SimscapeFilterOrder=2  InputFilterTimeConstant=0.001  UdotUserProvided=0
  Solver Configuration : nesl_utility/Solver Configuration  PhysicalDomain=network_engine_domain  SubClassName=solver  LeftPortType=input  RightPortType=generic  Tones=[]  Harmonics=[]  SimulateNoise=off  Profile=off  UseLocalSampling=off  EnableSwitchedLinearOptims=on  FrequencyDomain=off  UseCCode=off  RelTol=0.001  AbsTol=0.001  MinStep=1e-09  ToWorkspace=off  RevertToSquareIcSolve=off  NumHomotopyIterations=100  PhasorMode=off  PhasorModeNumHarmonics=1  ConsistencySolver=NEWTON_XTOL_AFTER_FTOL  IndexReductionMethod=DerivativeReplacement  DoDC=off  ResidualTolerance=1e-09  ConsistencyTolSource=GLOBAL  ConsistencyAbsTol=0.001  ConsistencyRelTol=0.001  ConsistencyTolFactor=0.001  UseLocalSolver=off  LocalSolverChoice=NE_BACKWARD_EULER_ADVANCER  ResolveIndetEquations=on  FunctionEvalNumThread=1  LocalSolverSampleTime=0.001  DoFixedCost=off  MaxNonlinIter=3  MaxModeIter=2  ComputeImpulses=off  ImpulseIterations=2  LinearAlgebra=auto  LinearAlgebraNumThread=0  EquationFormulation=NE_TIME_EF  DelaysMemoryBudget=1024  AutomaticFiltering=on  FilteringTimeConstant=0.001  PartitionStorageMethod=AS_NEEDED  PartitionMemoryBudget=1024  PartitionMethod=ROBUST  MultibodyUseLocalSolver=off  MultibodyLocalSolverChoice=ODE1  MultibodyLocalSolverSampleTime=0.001
  Solver Configuration2 : nesl_utility/Solver Configuration  PhysicalDomain=network_engine_domain  SubClassName=solver  LeftPortType=input  RightPortType=generic  Tones=[]  Harmonics=[]  SimulateNoise=off  Profile=off  UseLocalSampling=off  EnableSwitchedLinearOptims=on  FrequencyDomain=off  UseCCode=off  RelTol=0.001  AbsTol=0.001  MinStep=1e-09  ToWorkspace=off  RevertToSquareIcSolve=off  NumHomotopyIterations=100  PhasorMode=off  PhasorModeNumHarmonics=1  ConsistencySolver=NEWTON_XTOL_AFTER_FTOL  IndexReductionMethod=DerivativeReplacement  DoDC=off  ResidualTolerance=1e-09  ConsistencyTolSource=GLOBAL  ConsistencyAbsTol=0.001  ConsistencyRelTol=0.001  ConsistencyTolFactor=0.001  UseLocalSolver=off  LocalSolverChoice=NE_PARTITIONING_ADVANCER  ResolveIndetEquations=on  FunctionEvalNumThread=1  LocalSolverSampleTime=0.001  DoFixedCost=off  MaxNonlinIter=3  MaxModeIter=2  ComputeImpulses=off  ImpulseIterations=2  LinearAlgebra=auto  LinearAlgebraNumThread=0  EquationFormulation=NE_TIME_EF  DelaysMemoryBudget=1024  AutomaticFiltering=on  FilteringTimeConstant=0.001  PartitionStorageMethod=AS_NEEDED  PartitionMemoryBudget=1024  PartitionMethod=FAST  MultibodyUseLocalSolver=off  MultibodyLocalSolverChoice=ODE1  MultibodyLocalSolverSampleTime=0.001
  Spatial Contact Force : sm_lib/Forces and Torques/Spatial Contact Force  SenseSeparationDistance=off  NormalForceType=SmoothSpringDamper  NormalStiffness=1e6  NormalStiffnessUnits=N/m  NormalDamping=1.2e3  NormalDampingUnits=N/(m/s)  NormalTransitionRegionWidth=1e-4  NormalTransitionRegionWidthUnits=m  FrictionType=SmoothStickSlip  CoefficientOfStaticFriction=1.2  CoefficientOfDynamicFriction=0.7  FrictionalCriticalVelocity=1e-3  FrictionalCriticalVelocityUnits=m/s  SenseContactSignal=off  SensePenetrationDepth=off  SenseNormalVelocity=off  SenseTangentialVelocity=off  SensingForceTorqueDirection=BaseOnFollower  SensingForceTorqueResolutionFrame=ContactFrame  SenseNormalForce=off  SenseNormalForceMagnitude=off  SenseNormalTorque=off  SenseFrictionalForce=off  SenseFrictionalForceMagnitude=off  SenseFrictionalTorque=off  SenseTotalForce=off  SenseTotalTorque=off  SenseContactBaseRotation=off  SenseContactBaseTranslation=off  SenseContactFollowerRotation=off  SenseContactFollowerTranslation=off  ZeroCrossDetectContactStartAndEnd=off
  Spatial Contact Force1 : sm_lib/Forces and Torques/Spatial Contact Force  SenseSeparationDistance=off  NormalForceType=SmoothSpringDamper  NormalStiffness=1e6  NormalStiffnessUnits=N/m  NormalDamping=1.2e3  NormalDampingUnits=N/(m/s)  NormalTransitionRegionWidth=1e-4  NormalTransitionRegionWidthUnits=m  FrictionType=SmoothStickSlip  CoefficientOfStaticFriction=1.2  CoefficientOfDynamicFriction=0.7  FrictionalCriticalVelocity=1e-3  FrictionalCriticalVelocityUnits=m/s  SenseContactSignal=off  SensePenetrationDepth=off  SenseNormalVelocity=off  SenseTangentialVelocity=off  SensingForceTorqueDirection=BaseOnFollower  SensingForceTorqueResolutionFrame=ContactFrame  SenseNormalForce=off  SenseNormalForceMagnitude=off  SenseNormalTorque=off  SenseFrictionalForce=off  SenseFrictionalForceMagnitude=off  SenseFrictionalTorque=off  SenseTotalForce=off  SenseTotalTorque=off  SenseContactBaseRotation=off  SenseContactBaseTranslation=off  SenseContactFollowerRotation=off  SenseContactFollowerTranslation=off  ZeroCrossDetectContactStartAndEnd=off
  Step1 : Step  Time=6  After=-0.25  SampleTime=0
  Step3 : Step  After=-0.25  SampleTime=0
  Sum : Sum  Inputs=|+-
  Sum of Elements{1..4} (4 alike) : Sum  Inputs=+  CollapseMode=Specified dimension  CollapseDim=2
  Transfer Fcn : TransferFcn  Denominator=[1 1]
  Wheel L : sm_lib/Body Elements/Cylindrical Solid  CylinderRadius=robot_params.Rw*1.3  CylinderRadiusUnits=m  CylinderLength=0.05  CylinderLengthUnits=m  ExportEntireGeometry=on  InertiaType=Custom  BasedOnType=Density  Density=1000  DensityUnits=kg/m^3  Mass=robot_params.mw  MassUnits=kg  CenterOfMass=[0 0 0]  CenterOfMassUnits=m  MomentsOfInertia=[1.412017 1.412017 2.822575]  MomentsOfInertiaUnits=kg*m^2  ProductsOfInertia=[0 0 0]  ProductsOfInertiaUnits=kg*m^2  GraphicType=FromGeometry  MarkerShape=Sphere  MarkerSize=10  GraphicVisPropType=SimpleVisualProperties  GraphicDiffuseColor=[0.5 0.5 0.5]  GraphicOpacity=1  GraphicSpecularColor=[0.5 0.5 0.5 1.0]  GraphicAmbientColor=[0.15 0.15 0.15 1.0]  GraphicEmissiveColor=[0.0 0.0 0.0 1.0]  GraphicShininess=75  DoExposeReferenceFrame=on  SerializedFrames=<Frames/>
  Wheel L sensing : Subsystem
      settings: PortSchema="{\"entries\":[{\"content\":{\"sides\":[{\"content\":{},\"type\":\"ConnectorPlacement.EquallySpacedRectSide\",\"uuid\":\"ea9d79d0-a490-4652-82e6-557e12b0aba5\"},{\"content\":{\"side\":\"RIGHT\"},\"type\":\"ConnectorPlacement.EquallySpacedRectSide\",\"uuid\":\"f32903a1-4d8b-4407-8bbb-547edd3cb5f6\"},{\"content\":{\"side\":\"TOP\"},\"type\":\"ConnectorPlacement.EquallySpacedRectSide\",\"uuid\":\"fbee0b4d-6271-40ea-8dd1-d28f8c19f4ef\"},{\"content\":{\"connectorIds\":[\"RConn1\"],\"side\":\"BOTTOM\"},\"type\":\"ConnectorPlacement.EquallySpacedRectSide\",\"uuid\":\"cbab87b1-08d9-47a6-9493-a07b4ae6b609\"}]},\"type\":\"ConnectorPlacement.EquallySpacedConnector\",\"uuid\":\"a82548d1-a5fc-4c9c-b8a0-1d70df1cc0c8\"}],\"packageUris\":[\"http://schema.mathworks.com/mf0/Connector/R2020b\"],\"version\":\"1.0\"}"
  Wheel R : sm_lib/Body Elements/Cylindrical Solid  CylinderRadius=robot_params.Rw*1.3  CylinderRadiusUnits=m  CylinderLength=0.05  CylinderLengthUnits=m  ExportEntireGeometry=on  InertiaType=Custom  BasedOnType=Density  Density=1000  DensityUnits=kg/m^3  Mass=robot_params.mw  MassUnits=kg  CenterOfMass=[0 0 0]  CenterOfMassUnits=m  MomentsOfInertia=[1.412017 1.412017 2.822575]  MomentsOfInertiaUnits=kg*m^2  ProductsOfInertia=[0 0 0]  ProductsOfInertiaUnits=kg*m^2  GraphicType=FromGeometry  MarkerShape=Sphere  MarkerSize=10  GraphicVisPropType=SimpleVisualProperties  GraphicDiffuseColor=[0.5 0.5 0.5]  GraphicOpacity=1  GraphicSpecularColor=[0.5 0.5 0.5 1.0]  GraphicAmbientColor=[0.15 0.15 0.15 1.0]  GraphicEmissiveColor=[0.0 0.0 0.0 1.0]  GraphicShininess=75  DoExposeReferenceFrame=on  SerializedFrames=<Frames/>
  Wheel R sensing : Subsystem
      settings: PortSchema="{\"entries\":[{\"content\":{\"sides\":[{\"content\":{},\"type\":\"ConnectorPlacement.EquallySpacedRectSide\",\"uuid\":\"ea9d79d0-a490-4652-82e6-557e12b0aba5\"},{\"content\":{\"side\":\"RIGHT\"},\"type\":\"ConnectorPlacement.EquallySpacedRectSide\",\"uuid\":\"f32903a1-4d8b-4407-8bbb-547edd3cb5f6\"},{\"content\":{\"side\":\"TOP\"},\"type\":\"ConnectorPlacement.EquallySpacedRectSide\",\"uuid\":\"fbee0b4d-6271-40ea-8dd1-d28f8c19f4ef\"},{\"content\":{\"connectorIds\":[\"RConn1\"],\"side\":\"BOTTOM\"},\"type\":\"ConnectorPlacement.EquallySpacedRectSide\",\"uuid\":\"cbab87b1-08d9-47a6-9493-a07b4ae6b609\"}]},\"type\":\"ConnectorPlacement.EquallySpacedConnector\",\"uuid\":\"a82548d1-a5fc-4c9c-b8a0-1d70df1cc0c8\"}],\"packageUris\":[\"http://schema.mathworks.com/mf0/Connector/R2020b\"],\"version\":\"1.0\"}"
  World Frame : sm_lib/Frames and Transforms/World Frame
  World Frame1 : sm_lib/Frames and Transforms/World Frame
  World Frame3 : sm_lib/Frames and Transforms/World Frame
  World to Head : sm_lib/Frames and Transforms/Rigid Transform  RotationMethod=None  FollAlignAxisA=+X  BaseAlignAxisA=+Y  FollAlignAxisB=+Y  BaseAlignAxisB=+Z  RotationStandardAxis=+Z  RotationAngle=0  RotationAngleUnits=deg  RotationArbitraryAxis=[0 0 1]  RotationSequenceAxes=FollowerAxes  RotationSequence=XYX  RotationSequenceAngles=[0 0 0]  RotationSequenceAnglesUnits=deg  RotationMatrix=[1 0 0;0 1 0;0 0 1]  Quaternion=[1 0 0 0]  TranslationMethod=Cartesian  TranslationCartesianOffset=[0 0 1.25]  TranslationCartesianOffsetUnits=m  TranslationStandardAxis=+Z  TranslationStandardOffset=0  TranslationStandardOffsetUnits=m  TranslationROffset=0  TranslationROffsetUnits=m  TranslationThetaOffset=0  TranslationThetaOffsetUnits=deg  TranslationZOffset=0  TranslationZOffsetUnits=m
  Zero : Constant  Value=0  OutDataTypeStr=Inherit: Inherit via back propagation
  Zero-Order Hold2 : ZeroOrderHold  SampleTime=Ts
  Zero-Order Hold3 : ZeroOrderHold  SampleTime=Ts
  Zero2 : Constant  Value=[pi/3;-pi/6]  OutDataTypeStr=Inherit: Inherit via back propagation
  center : sm_lib/Joints/Cartesian Joint  JointMode=Normal  CompositeWrenchDir=FollowerOnBase  CompositeWrenchFrame=BaseFrame  SenseConstraintForce=off  SenseConstraintTorque=off  SenseTotalForce=off  SenseTotalTorque=off  PxPositionTargetSpecify=off  PxPositionTargetPriority=High  PxPositionTargetValue=0  PxPositionTargetValueUnits=m  PxVelocityTargetSpecify=off  PxVelocityTargetPriority=High  PxVelocityTargetValue=0  PxVelocityTargetValueUnits=m/s  PxEquilibriumPosition=0  PxEquilibriumPositionUnits=m  PxSpringStiffness=0  PxSpringStiffnessUnits=N/m  PxDampingCoefficient=0  PxDampingCoefficientUnits=N/(m/s)  PxLowerLimitSpecify=off  PxLowerLimitBound=-1  PxLowerLimitBoundUnits=m  PxLowerLimitStiffness=1e6  PxLowerLimitStiffnessUnits=N/m  PxLowerLimitDamping=1e3  PxLowerLimitDampingUnits=N/(m/s)  PxLowerLimitTransitionRegionWidth=1e-4  PxLowerLimitTransitionRegionWidthUnits=m  PxUpperLimitSpecify=off  PxUpperLimitBound=1  PxUpperLimitBoundUnits=m  PxUpperLimitStiffness=1e6  PxUpperLimitStiffnessUnits=N/m  PxUpperLimitDamping=1e3  PxUpperLimitDampingUnits=N/(m/s)  PxUpperLimitTransitionRegionWidth=1e-4  PxUpperLimitTransitionRegionWidthUnits=m  PxTorqueActuationMode=ComputedTorque  PxMotionActuationMode=InputMotion  PxSensePosition=off  PxSenseVelocity=off  PxSenseAcceleration=off  PxSenseTorqueForce=off  PxSenseLowerLimitTorqueForce=off  PxSenseUpperLimitTorqueForce=off  PyPositionTargetSpecify=off  PyPositionTargetPriority=High  PyPositionTargetValue=0  PyPositionTargetValueUnits=m  PyVelocityTargetSpecify=off  PyVelocityTargetPriority=High  PyVelocityTargetValue=0  PyVelocityTargetValueUnits=m/s  PyEquilibriumPosition=0  PyEquilibriumPositionUnits=m  PySpringStiffness=0  PySpringStiffnessUnits=N/m  PyDampingCoefficient=0  PyDampingCoefficientUnits=N/(m/s)  PyLowerLimitSpecify=off  PyLowerLimitBound=-1  PyLowerLimitBoundUnits=m  PyLowerLimitStiffness=1e6  PyLowerLimitStiffnessUnits=N/m  PyLowerLimitDamping=1e3  PyLowerLimitDampingUnits=N/(m/s)  PyLowerLimitTransitionRegionWidth=1e-4  PyLowerLimitTransitionRegionWidthUnits=m  PyUpperLimitSpecify=off  PyUpperLimitBound=1  PyUpperLimitBoundUnits=m  PyUpperLimitStiffness=1e6  PyUpperLimitStiffnessUnits=N/m  PyUpperLimitDamping=1e3  PyUpperLimitDampingUnits=N/(m/s)  PyUpperLimitTransitionRegionWidth=1e-4  PyUpperLimitTransitionRegionWidthUnits=m  PyTorqueActuationMode=ComputedTorque  PyMotionActuationMode=InputMotion  PySensePosition=off  PySenseVelocity=off  PySenseAcceleration=off  PySenseTorqueForce=off  PySenseLowerLimitTorqueForce=off  PySenseUpperLimitTorqueForce=off  PzPositionTargetSpecify=off  PzPositionTargetPriority=High  PzPositionTargetValue=0  PzPositionTargetValueUnits=m  PzVelocityTargetSpecify=off  PzVelocityTargetPriority=High  PzVelocityTargetValue=0  PzVelocityTargetValueUnits=m/s  PzEquilibriumPosition=0  PzEquilibriumPositionUnits=m  PzSpringStiffness=0  PzSpringStiffnessUnits=N/m  PzDampingCoefficient=0  PzDampingCoefficientUnits=N/(m/s)  PzLowerLimitSpecify=off  PzLowerLimitBound=-1  PzLowerLimitBoundUnits=m  PzLowerLimitStiffness=1e6  PzLowerLimitStiffnessUnits=N/m  PzLowerLimitDamping=1e3  PzLowerLimitDampingUnits=N/(m/s)  PzLowerLimitTransitionRegionWidth=1e-4  PzLowerLimitTransitionRegionWidthUnits=m  PzUpperLimitSpecify=off  PzUpperLimitBound=1  PzUpperLimitBoundUnits=m  PzUpperLimitStiffness=1e6  PzUpperLimitStiffnessUnits=N/m  PzUpperLimitDamping=1e3  PzUpperLimitDampingUnits=N/(m/s)  PzUpperLimitTransitionRegionWidth=1e-4  PzUpperLimitTransitionRegionWidthUnits=m  PzTorqueActuationMode=ComputedTorque  PzMotionActuationMode=InputMotion  PzSensePosition=off  PzSenseVelocity=off  PzSenseAcceleration=off  PzSenseTorqueForce=off  PzSenseLowerLimitTorqueForce=off  PzSenseUpperLimitTorqueForce=off
  center sensing : Subsystem
      settings: PortSchema="{\"entries\":[{\"content\":{\"sides\":[{\"content\":{\"connectorIds\":[\"LConn1\"]},\"type\":\"ConnectorPlacement.EquallySpacedRectSide\",\"uuid\":\"a482bcdd-5ef2-44be-8ef1-888cdf1c267b\"},{\"content\":{\"connectorIds\":[\"RConn1\"],\"side\":\"RIGHT\"},\"type\":\"ConnectorPlacement.EquallySpacedRectSide\",\"uuid\":\"327854d7-5112-4707-805d-1470fb22930d\"},{\"content\":{\"side\":\"TOP\"},\"type\":\"ConnectorPlacement.EquallySpacedRectSide\",\"uuid\":\"7fa4ba6c-99fc-4aa9-8971-707b95549c0c\"},{\"content\":{\"connectorIds\":[\"RConn2\"],\"side\":\"BOTTOM\"},\"type\":\"ConnectorPlacement.EquallySpacedRectSide\",\"uuid\":\"86643d71-4cd3-4215-a6cf-4ad6925abbeb\"}]},\"type\":\"ConnectorPlacement.EquallySpacedConnector\",\"uuid\":\"2f0e97e0-ec09-4e22-9388-9e9e2b3106c7\"}],\"packageUris\":[\"http://schema.mathworks.com/mf0/Connector/R2020b\"],\"version\":\"1.0\"}"
  center_vis : sm_lib/Body Elements/Brick Solid  BrickDimensions=[.05 .05 .05]  BrickDimensionsUnits=m  ExportEntireGeometry=off  InertiaType=PointMass  BasedOnType=Density  Density=1000  DensityUnits=kg/m^3  Mass=0.001  MassUnits=kg  CenterOfMass=[0 0 0]  CenterOfMassUnits=m  MomentsOfInertia=[1 1 1]  MomentsOfInertiaUnits=kg*m^2  ProductsOfInertia=[0 0 0]  ProductsOfInertiaUnits=kg*m^2  GraphicType=FromGeometry  MarkerShape=Sphere  MarkerSize=10  GraphicVisPropType=SimpleVisualProperties  GraphicDiffuseColor=[0 0 0]  GraphicOpacity=1  GraphicSpecularColor=[0.5 0.5 0.5 1.0]  GraphicAmbientColor=[0.15 0.15 0.15 1.0]  GraphicEmissiveColor=[0.0 0.0 0.0 1.0]  GraphicShininess=75  DoExposeReferenceFrame=on  SerializedFrames=<Frames/>
  ddq : Scope  Commented=on  NumInputPorts=6
      settings: ActiveDisplayString=3  Title=ddq Knee-Wheel R  ActiveDisplayYMinimum=-928.0590914997897  ActiveDisplayYMaximum=1275.6754291952052  DataLoggingVariableName=ScopeData2
  dq : Scope  Commented=on  NumInputPorts=6
      settings: ActiveDisplayString=3  Title=dq Knee-Wheel R  ActiveDisplayYMinimum=-0.1012611394776765  ActiveDisplayYMaximum=0.56881503276014012
  q : Scope  Commented=on  NumInputPorts=6
      settings: ActiveDisplayString=3  Title=q Knee-Wheel R  ActiveDisplayYMinimum=-4.0705502548513239  ActiveDisplayYMaximum=32.9979718473207
  tau : Scope  Commented=on  NumInputPorts=6
      settings: Title="tau Head-Hip R  Joint"  ActiveDisplayYMinimum=-181.05320578285196  ActiveDisplayYMaximum=75.195564403256611  DataLoggingVariableName=ScopeData3
  wires:
  Demux/1 -> q/1
  Demux/2 -> q/2
  Demux/3 -> q/3
  Demux/4 -> q/4
  Demux/5 -> q/5
  Demux/6 -> q/6
  Data Store Read/1 -> Demux/1
  Data Store Read1/1 -> Demux1/1
  Demux1/5 -> dq/5
  Demux1/4 -> dq/4
  Demux1/3 -> dq/3
  Demux1/2 -> dq/2
  Demux1/1 -> dq/1
  Demux1/6 -> dq/6
  Demux2/6 -> ddq/6
  Demux2/1 -> ddq/1
  Demux2/2 -> ddq/2
  Demux2/3 -> ddq/3
  Demux2/4 -> ddq/4
  Demux2/5 -> ddq/5
  Data Store Read2/1 -> Demux2/1
  Data Store Read3/1 -> Demux3/1
  Demux3/6 -> tau/6
  Demux3/5 -> tau/5
  Demux3/4 -> tau/4
  Demux3/3 -> tau/3
  Demux3/2 -> tau/2
  Demux3/1 -> tau/1
  Constant1/1 -> Data Store Write2/1
  Constant2/1 -> [h_des]
  Data Store Read14/1 -> Mux4/1
  Data Store Read15/1 -> Mux4/2
  Mux4/1 -> Scope2/1
  Data Store Read16/1 -> Scope2/2
  Data Store Read18/1 -> Mux5/2
  Data Store Read17/1 -> Mux5/1
  Mux5/1 -> Scope2/3
  Data Store Read19/1 -> Scope2/4
  Mux6/1 -> Scope2/5
  Data Store Read22/1 -> Scope2/6
  Data Store Read21/1 -> Mux6/2
  Data Store Read20/1 -> Mux6/1
  Data Store Read24/1 -> Mux7/1
  Data Store Read25/1 -> Mux7/2
  Mux7/1 -> Scope2/7
  Data Store Read26/1 -> Scope2/8
  [wx] -> Scope/2
  Data Store Read10/1 -> Scope/4
  Data Store Read11/1 -> Gain/1
  Gain/1 -> Scope1/1
  Clock2/1 -> MATLAB Function3/1(t)
  MATLAB Function3/2(s_dot_des) -> [s_dot_des]
  Gain17/1 -> [CoM_p]
  Matrix Concatenate1/1 -> Sum of Elements1/1
  Demux4/1 -> Simulink-PS Converter1/1
  Demux4/2 -> Simulink-PS Converter2/1
  Demux4/3 -> Simulink-PS Converter3/1
  [CoM_p] -> Demux4/1
  [center_p] -> Demux5/1
  Demux5/2 -> Simulink-PS Converter5/1
  Demux5/1 -> Simulink-PS Converter4/1
  Demux5/3 -> Simulink-PS Converter6/1
  Gain11/1 -> Matrix Concatenate2/5
  Gain10/1 -> Matrix Concatenate2/4
  Gain9/1 -> Matrix Concatenate2/3
  Gain8/1 -> Matrix Concatenate2/2
  Gain7/1 -> Matrix Concatenate2/1
  Matrix Concatenate2/1 -> Sum of Elements2/1
  Gain12/1 -> [CoM_v]
  Sum of Elements2/1 -> Gain12/1
  Selector11/1 -> Gain11/1
  Selector10/1 -> Gain10/1
  Selector9/1 -> Gain9/1
  Selector8/1 -> Gain8/1
  Selector7/1 -> Gain7/1
  Data Store Read13/1 -> Selector10/1, Selector11/1, Selector9/1, Selector7/1, Selector8/1
  [UB_p] -> MATLAB Function4/1(CoM_p)
  [center_p] -> MATLAB Function4/2(center_p)
  [UB_v] -> MATLAB Function4/3(CoM_v)
  [center_v] -> MATLAB Function4/4(center_v)
  MATLAB Function3/1(s_des) -> [s_des]
  [CoM_v] -> Selector13/1
  Selector13/1 -> Mux2/1
  [s_dot_des] -> Mux2/2
  Mux2/1 -> Scope/3
  [alpha] -> Mux8/1
  Mux8/1 -> Scope/1
  Data Store Read4/1 -> Demux6/1
  Demux6/2 -> [q2_R]
  Demux7/2 -> [q2_L]
  Demux6/3 -> [qw_R]
  Demux6/1 -> [q3_R]
  Data Store Read8/1 -> Demux7/1
  Demux7/1 -> [q3_L]
  Demux7/3 -> [qw_L]
  [q3_R] -> Mux/3
  [qw_R] -> Mux/2
  [q2_R] -> Mux/1
  [dq1_R] -> Mux1/2
  Data Store Read5/1 -> Mux1/1
  Data Store Read6/1 -> Mux9/1
  [dq1_L] -> Mux9/2
  [q2_L] -> Mux3/1
  [qw_L] -> Mux3/2
  [q3_L] -> Mux3/3
  [q1_L] -> Mux3/4
  Selector14/1 -> [dq1_L], [dq1_R]
  [w_Head] -> Selector14/1
  [v_wheel_L] -> Gain13/1
  Gain13/1 -> Matrix Concatenate2/6
  [v_wheel_R] -> Gain14/1
  Gain14/1 -> Matrix Concatenate2/7
  Selector5/1 -> Gain15/1
  Selector6/1 -> Gain16/1
  Selector3/1 -> Gain2/1
  Selector2/1 -> Gain1/1
  Gain1/1 -> Matrix Concatenate1/4
  Gain5/1 -> Matrix Concatenate1/1
  Gain4/1 -> Matrix Concatenate1/7
  Gain3/1 -> Matrix Concatenate1/6
  [p_wheel_R] -> Gain4/1
  Data Store Read12/1 -> Selector4/1, Selector5/1, Selector2/1, Selector3/1, Selector6/1
  Gain15/1 -> Matrix Concatenate1/2
  Gain16/1 -> Matrix Concatenate1/3
  Selector4/1 -> Gain5/1
  [p_wheel_L] -> Gain3/1
  Gain2/1 -> Matrix Concatenate1/5
  Sum of Elements1/1 -> Gain17/1
  [q1_R] -> Mux/4
  MATLAB Function4/1(alpha) -> Gain6/1
  Gain6/1 -> [alpha]
  MATLAB Function4/2(wx) -> Gain18/1
  Gain18/1 -> [wx]
  Mux/1 -> [Q_R]
  [Q_R] -> MATLAB Function5/1(Q_R)
  Mux1/1 -> [dQ_R]
  [dQ_R] -> MATLAB Function5/2(dQ_R)
  Mux3/1 -> [Q_L]
  Mux9/1 -> [dQ_L]
  [dQ_L] -> MATLAB Function5/4(dQ_L)
  [Q_L] -> MATLAB Function5/3(Q_L)
  MATLAB Function5/3(dIv) -> Integrator4/1
  MATLAB Function5/4(dW) -> Integrator5/1
  [wx] -> MATLAB Function5/7(dth_meas)
  [CoM_v] -> Selector20/1  "CoM_v"
  Selector20/1 -> MATLAB Function5/8(v_meas)  "CoM_vx"
  Selector21/1 -> [q1_R], [q1_L]
  [seq_Head] -> Selector21/1
  Demux9/1 -> Scope5/1
  Demux9/2 -> Scope5/2
  Data Store Read7/1 -> Demux9/1
  Data Store Read23/1 -> Scope8/1
  [err_theta] -> Scope8/3
  Data Store Read27/1 -> Scope8/4
  [alpha] -> Scope9/1
  [wx] -> Scope9/2
  MATLAB Function5/6(th_ref) -> [theta_ref]
  Mux12/1 -> Scope8/2
  [theta_ref] -> Mux12/2
  [alpha] -> Mux12/1
  MATLAB Function5/2(tau_L) -> Zero-Order Hold3/1
  MATLAB Function5/1(tau_R) -> Zero-Order Hold2/1
  Data Store Read28/1 -> Selector23/1
  Data Store Read9/1 -> Selector24/1
  [alpha] -> MATLAB Function5/6(th_meas)
  Mux10/1 -> Data Store Write4/1
  From30/1 -> Gain19/1
  Gain19/1 -> Mux10/1, Mux10/2
  Integrator5/1 -> [W]
  Integrator4/1 -> [Iv]
  [Iv] -> MATLAB Function5/10(Iv)
  [W] -> MATLAB Function5/11(W)
  [theta_ref] -> Mux8/2
  MATLAB Function5/7(err_theta) -> [err_theta]
  [Qref] -> MATLAB Function5/5(Q_ref)
  Mux13/1 -> Data Store Write3/1
  Zero-Order Hold2/1 -> [tau_R]
  Zero-Order Hold3/1 -> [tau_L]
  [tau_L] -> Data Store Write1/1
  [tau_R] -> Data Store Write/1
  Zero2/1 -> [Qref]
  Sum of Elements3/1 -> Gain28/1
  Gain29/1 -> Matrix Concatenate3/5
  Selector18/1 -> Gain32/1
  Gain27/1 -> Matrix Concatenate3/3
  Gain26/1 -> Matrix Concatenate3/2
  Data Store Read29/1 -> Selector22/1, Selector17/1, Selector16/1, Selector19/1, Selector18/1
  Gain32/1 -> Matrix Concatenate3/1
  Gain20/1 -> Matrix Concatenate3/4
  Selector16/1 -> Gain20/1
  Selector17/1 -> Gain29/1
  Selector22/1 -> Gain27/1
  Selector19/1 -> Gain26/1
  Data Store Read30/1 -> Selector26/1, Selector25/1, Selector27/1, Selector12/1, Selector15/1
  Selector25/1 -> Gain33/1
  Selector26/1 -> Gain34/1
  Selector27/1 -> Gain35/1
  Selector12/1 -> Gain21/1
  Selector15/1 -> Gain22/1
  Sum of Elements4/1 -> Gain23/1
  Gain23/1 -> [UB_v]
  Matrix Concatenate4/1 -> Sum of Elements4/1
  Gain33/1 -> Matrix Concatenate4/1
  Gain34/1 -> Matrix Concatenate4/2
  Gain35/1 -> Matrix Concatenate4/3
  Gain21/1 -> Matrix Concatenate4/4
  Gain22/1 -> Matrix Concatenate4/5
  Matrix Concatenate3/1 -> Sum of Elements3/1
  Gain28/1 -> [UB_p]
  Selector/1 -> Mux14/1
  Zero/1 -> Mux14/2
  Mux14/1 -> Mux13/2, Mux13/1
  [Qref] -> Selector/1
  Data Store Read36/1 -> Scope4/4
  Mux15/1 -> Scope4/3
  Data Store Read34/1 -> Mux15/1
  Data Store Read35/1 -> Mux15/2
  Data Store Read33/1 -> Scope4/2
  Mux11/1 -> Scope4/1
  Data Store Read32/1 -> Mux11/2
  Data Store Read31/1 -> Mux11/1
  [alpha] -> Mux16/1
  [theta_ref] -> Mux16/2
  Mux16/1 -> Scope4/6
  Data Store Read37/1 -> Scope4/8
  [CoM_v] -> Selector1/1
  [vref] -> MATLAB Function5/9(v_ref)
  Mux17/1 -> Scope4/5
  Selector1/1 -> Mux17/1
  [vref] -> Mux17/2
  Repeating Sequence/1 -> [vref]
  Step1/1 -> Sum/2
  Step3/1 -> Sum/1
  Sum/1 -> Transfer Fcn/1
  [CoM_p] -> Selector28/1
  Selector28/1 -> Scope4/7
  connections:
  World Frame/RConn1 -- Gravity/RConn1 -- World to Head/LConn1 -- Head Sensing/RConn1 -- Solver Configuration/RConn1
  6-DOF Joint/RConn1 -- "Head to Head-Hip R  "/LConn1 -- Head/RConn1 -- "Head to Head-Hip L "/LConn1 -- Head Sensing/LConn1
  "Hip to HIP-Knee R "/LConn1 -- Hip R sensing/RConn1 -- Hip R/RConn1 -- Head-Hip to Hip R/RConn1
  Knee R/RConn1 -- Knee R sensing/RConn1 -- "Knee to Knee-Wheel R "/LConn1 -- Hip-Knee to Knee R/RConn1
  Infinite Plane/LConn1 -- center sensing/RConn2 -- World Frame1/RConn1
  World to Head/RConn1 -- 6-DOF Joint/LConn1
  Spatial Contact Force/LConn1 -- Wheel L/LConn1
  Spatial Contact Force1/LConn1 -- Wheel R/LConn1
  Hip to Hip-Knee L/LConn1 -- Hip L sensing/RConn1 -- Hip L/RConn1 -- Head-Hip to Hip L/RConn1
  Knee to Knee-Wheel L/LConn1 -- Knee R1/RConn1 -- Knee L sensing/RConn1 -- Hip-Knee to Knee L/RConn1
  "Head to Head-Hip R  "/RConn1 -- "Head-Hip R Joint "/LConn1
  Head-Hip to Hip R/LConn1 -- "Head-Hip R Joint "/RConn1
  "Head to Head-Hip L "/RConn1 -- "Head-Hip L Joint "/LConn1
  Head-Hip to Hip L/LConn1 -- "Head-Hip L Joint "/RConn1
  Hip-Knee R Joint/LConn1 -- "Hip to HIP-Knee R "/RConn1
  Hip-Knee to Knee R/LConn1 -- Hip-Knee R Joint/RConn1
  Knee-Wheel R Joint/LConn1 -- "Knee to Knee-Wheel R "/RConn1
  Knee-Wheel R Joint/RConn1 -- Wheel R sensing/RConn1 -- Wheel R/RConn1 -- center sensing/RConn1
  Hip to Hip-Knee L/RConn1 -- Hip-Knee L Joint/LConn1
  Hip-Knee to Knee L/LConn1 -- Hip-Knee L Joint/RConn1
  Knee-Wheel L Joint/LConn1 -- Knee to Knee-Wheel L/RConn1
  Knee-Wheel L Joint/RConn1 -- center sensing/LConn1 -- Wheel L/RConn1 -- Wheel L sensing/RConn1
  CoM/RConn1 -- CoM_vis/RConn1
  CoM/LConn4 -- Simulink-PS Converter3/RConn1
  CoM/LConn3 -- Simulink-PS Converter2/RConn1
  CoM/LConn2 -- Simulink-PS Converter1/RConn1
  Simulink-PS Converter4/RConn1 -- center/LConn2
  Simulink-PS Converter5/RConn1 -- center/LConn3
  Simulink-PS Converter6/RConn1 -- center/LConn4
  Infinite Plane/RConn1 -- Spatial Contact Force/RConn1 -- Spatial Contact Force1/RConn1
  center_vis/RConn1 -- center/RConn1
  Solver Configuration2/RConn1 -- CoM/LConn1 -- World Frame3/RConn1 -- center/LConn1
